simulink model "QPSK_TX_Final"  (R2017b)
settings: Solver=FixedStepDiscrete  StartTime=0.0  StopTime=1  RelTol=1e-3
PreLoadFcn:
  | qpsktxhdl=QPSK_final_init;
libraries: hdlsllib x3, dspmlti4 x2, commdigbbndpm3 x1
settings Model: DataTypeOverride=Off  Creator=The MathWorks, Inc.  LastModifiedBy=ppradhan
settings DataIOCC: LimitDataPoints=on  SaveFormat=Array  SaveOutput=off  SaveTime=off
settings OptimizationCC: BlockReduction=off  ConditionallyExecuteInputs=off  DefaultParameterBehavior=Inlined  LifeSpan=inf
settings DebuggingCC: AlgebraicLoopMsg=error  UnderspecifiedInitializationDetection=Classic  MergeDetectMultiDrivingBlocksExec=none  SolverPrmCheckMsg=warning  MultiTaskDSMMsg=warning  MultiTaskCondExecSysMsg=none  SingleTaskRateTransMsg=error  IntegerOverflowMsg=none  ParameterPrecisionLossMsg=none  AllowSymbolicDim=off  StateNameClashWarn=warning  SFUnexpectedBacktrackingDiag=warning  SFNoUnconditionalDefaultTransitionDiag=warning  SFExecutionAtInitializationDiag=none  IntegerSaturationMsg=none
settings HardwareCC: ProdBitPerPointer=32  ProdBitPerSizeT=32  ProdBitPerPtrDiffT=32  ProdLargestAtomicFloat=None  ProdIntDivRoundTo=Undefined  ProdEndianess=Unspecified  ProdWordSize=32  ProdHWDeviceType=ASIC/FPGA->ASIC/FPGA  ProdEqTarget=off
settings ModelReferenceCC: PropagateSignalLabelsOutOfModel=off
settings CodeAppCC: StateflowObjectComments=on
settings GRTTargetCC: TargetLangStandard=C89/C90 (ANSI)  GeneratePreprocessorConditionals=Disable all
settings ConfigComp: CovMetricSettings=dw  CovHtmlReporting=on  CovSaveCumulativeToWorkspaceVar=on  CovSaveSingleToWorkspaceVar=on  CovExternalEMLEnable=off  CovSFcnEnable=off

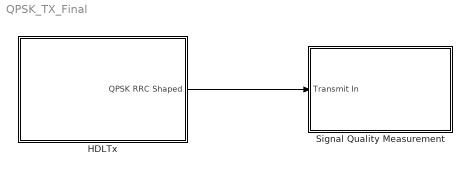
== system QPSK_TX_Final ==
  HDLTx : Subsystem
  Signal Quality Measurement : Subsystem
  wires:
  HDLTx/1(QPSK RRC Shaped) -> Signal Quality Measurement/1(Transmit In)

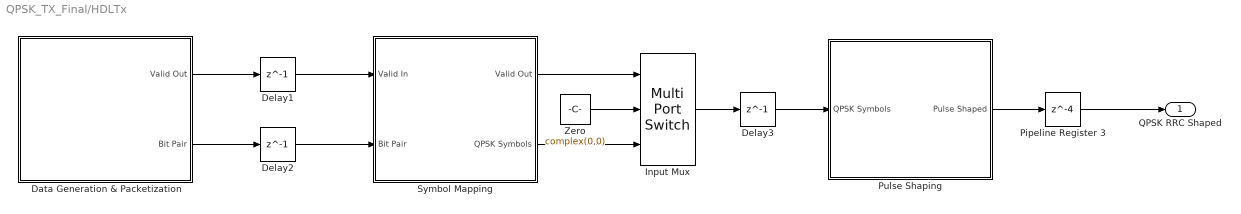
== system QPSK_TX_Final/HDLTx ==
  " Zero" : Constant  Value=complex(0,0)  OutDataTypeStr=fixdt(1,16,15)  SampleTime=(qpsktxhdl.Ts)*4
  Data Generation & Packetization : Subsystem
  Delay1 : Delay  DelayLength=1  InitialCondition=0
  Delay2 : Delay  DelayLength=1  InitialCondition=0
  Delay3 : Delay  DelayLength=1  InitialCondition=0
  Input Mux : MultiPortSwitch  DataPortOrder=Zero-based contiguous  Inputs=2
  Pipeline Register 3 : Delay  DelayLength=4  InitialCondition=0
  Pulse Shaping : Subsystem
  Symbol Mapping : Subsystem
  QPSK RRC Shaped : Outport
  wires:
  " Zero"/1 -> Input Mux/2
  Symbol Mapping/2(QPSK Symbols) -> Input Mux/3
  Symbol Mapping/1(Valid Out) -> Input Mux/1
  Delay3/1 -> Pulse Shaping/1(QPSK Symbols)
  Input Mux/1 -> Delay3/1
  Delay1/1 -> Symbol Mapping/1(Valid In)
  Pulse Shaping/1(Pulse Shaped) -> Pipeline Register 3/1
  Data Generation & Packetization/1(Valid Out) -> Delay1/1
  Pipeline Register 3/1 -> QPSK RRC Shaped/1
  Data Generation & Packetization/2(Bit Pair) -> Delay2/1
  Delay2/1 -> Symbol Mapping/2(Bit Pair)

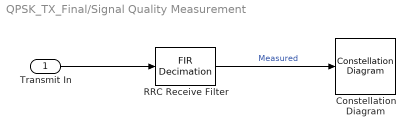
== system QPSK_TX_Final/Signal Quality Measurement ==
  Transmit In : Inport
  Constellation Diagram : ConstellationDiagram
  RRC Receive Filter : dspmlti4/FIR Decimation  FilterSource=Dialog parameters  h=qpsktxhdl.rcRxFilt  D=qpsktxhdl.Upsampling  filtStruct=Direct form  FilterObject=Hm_firdecim  framing=Allow multirate processing  inputOffset=0  outputBufInitCond=0  roundingMode=Floor  overflowMode=off  firstCoeffMode=Binary point scaling  firstCoeffWordLength=16  firstCoeffFracLength=15  firstCoeffDataTypeStr=fixdt(1,16,15)  firstCoeffMin=[]  firstCoeffMax=[]  firstCoeffLastDataTypeStr=fixdt(1,16,15)  prodOutputMode=Binary point scaling  prodOutputWordLength=32  prodOutputFracLength=30  prodOutputDataTypeStr=fixdt(1,32,30)  prodOutputLastDataTypeStr=fixdt(1,32,30)  accumMode=Binary point scaling  accumWordLength=33  accumFracLength=30  accumDataTypeStr=fixdt(1,33,30)  accumLastDataTypeStr=fixdt(1,33,30)  outputMode=Binary point scaling  outputWordLength=33  outputFracLength=30  outputDataTypeStr=fixdt(1,33,30)  outputMin=[]  outputMax=[]  outputLastDataTypeStr=fixdt(1,33,30)
  wires:
  Transmit In/1 -> RRC Receive Filter/1
  RRC Receive Filter/1 -> Constellation Diagram/1  "Measured"

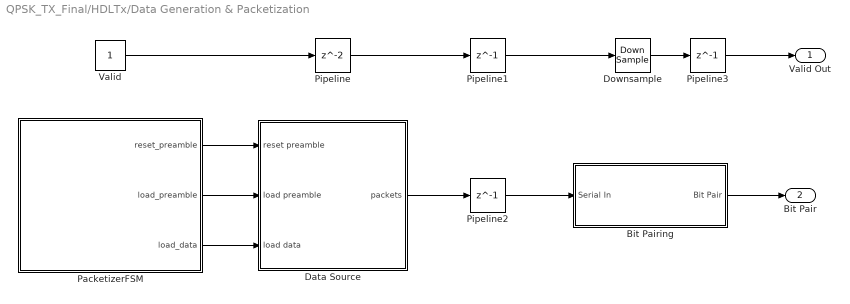
== system QPSK_TX_Final/HDLTx/Data Generation & Packetization ==
  Bit Pairing : Subsystem
  Data Source : Subsystem
  Downsample : DownSample  RateOptions=Allow multirate processing
  PacketizerFSM : MATLAB Function  TreatAsAtomicUnit=on  SystemSampleTime=(qpsktxhdl.Ts)*2
  Pipeline : Delay  InitialCondition=0
  Pipeline1 : Delay  DelayLength=1  InitialCondition=0
  Pipeline2 : Delay  DelayLength=1  InitialCondition=0
  Pipeline3 : Delay  DelayLength=1  InitialCondition=0
  Valid : Constant  OutDataTypeStr=boolean  SampleTime=(qpsktxhdl.Ts)*2
  Valid Out : Outport
  Bit Pair : Outport  Port=2
  wires:
  Bit Pairing/1(Bit Pair) -> Bit Pair/1
  Pipeline2/1 -> Bit Pairing/1(Serial In)
  Data Source/1(packets) -> Pipeline2/1
  Valid/1 -> Pipeline/1
  Pipeline1/1 -> Downsample/1
  Pipeline/1 -> Pipeline1/1
  Downsample/1 -> Pipeline3/1
  Pipeline3/1 -> Valid Out/1
  PacketizerFSM/1(reset_preamble) -> Data Source/1(reset preamble)
  PacketizerFSM/2(load_preamble) -> Data Source/2(load preamble)
  PacketizerFSM/3(load_data) -> Data Source/3(load data)

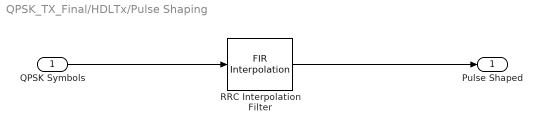
== system QPSK_TX_Final/HDLTx/Pulse Shaping ==
  QPSK Symbols : Inport
  RRC Interpolation Filter : dspmlti4/FIR Interpolation  FilterSource=Dialog parameters  h=qpsktxhdl.rcTxFilt  L=qpsktxhdl.Upsampling  FilterObject=Htxrc  framing=Allow multirate processing  outputBufInitCond=0  roundingMode=Floor  overflowMode=off  firstCoeffMode=Binary point scaling  firstCoeffWordLength=16  firstCoeffFracLength=15  firstCoeffDataTypeStr=fixdt(1,16,15)  firstCoeffMin=[]  firstCoeffMax=[]  firstCoeffLastDataTypeStr=fixdt(1,16,15)  prodOutputMode=Binary point scaling  prodOutputWordLength=16  prodOutputFracLength=15  prodOutputDataTypeStr=fixdt(1,16,15)  prodOutputLastDataTypeStr=fixdt(1,16,15)  accumMode=Binary point scaling  accumWordLength=16  accumFracLength=15  accumDataTypeStr=fixdt(1,16,15)  accumLastDataTypeStr=fixdt(1,16,15)  outputMode=Binary point scaling  outputWordLength=16  outputFracLength=15  outputDataTypeStr=fixdt(1,16,15)  outputMin=[]  outputMax=[]  outputLastDataTypeStr=fixdt(1,16,15)
      settings: SourceProductName=DSP System Toolbox
  Pulse Shaped : Outport
  wires:
  RRC Interpolation Filter/1 -> Pulse Shaped/1
  QPSK Symbols/1 -> RRC Interpolation Filter/1

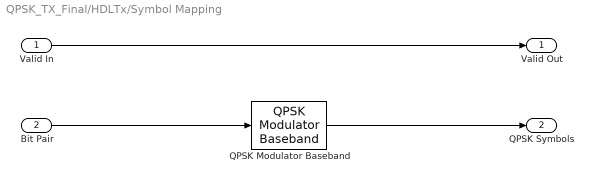
== system QPSK_TX_Final/HDLTx/Symbol Mapping ==
  Valid In : Inport
  Bit Pair : Inport  Port=2
  QPSK Modulator Baseband : commdigbbndpm3/QPSK Modulator Baseband  InType=Integer  Enc=Gray  Ph=pi/4  outDtype=Fixed-point  outWordLen=2  outUDDataType=sfix(16)  outFracLenMode=User-defined  outFracLen=0  outDataTypeStr=fixdt(1,2,0)  outLastDataTypeStr=fixdt(1,2,0)
  Valid Out : Outport
  QPSK Symbols : Outport  Port=2
  wires:
  Valid In/1 -> Valid Out/1
  Bit Pair/1 -> QPSK Modulator Baseband/1
  QPSK Modulator Baseband/1 -> QPSK Symbols/1

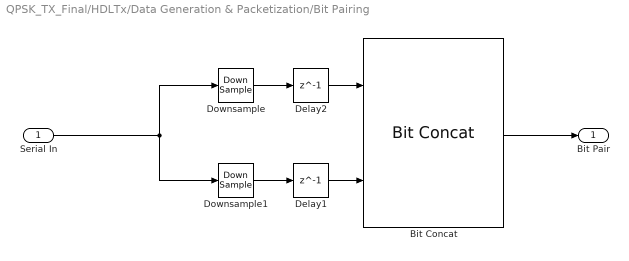
== system QPSK_TX_Final/HDLTx/Data Generation & Packetization/Bit Pairing ==
  Serial In : Inport
  Bit Concat : hdlsllib/HDL Operations/Bit Concat  numInputs=2
      settings: SourceProductName=HDL Coder  SourceProductBaseCode=HD
  Delay1 : Delay  DelayLength=1
  Delay2 : Delay  DelayLength=1
  Downsample : DownSample  phase=1  RateOptions=Allow multirate processing
  Downsample1 : DownSample  RateOptions=Allow multirate processing
  Bit Pair : Outport
  wires:
  Downsample1/1 -> Delay1/1
  Serial In/1 -> Downsample1/1, Downsample/1
  Bit Concat/1 -> Bit Pair/1
  Downsample/1 -> Delay2/1
  Delay1/1 -> Bit Concat/2
  Delay2/1 -> Bit Concat/1

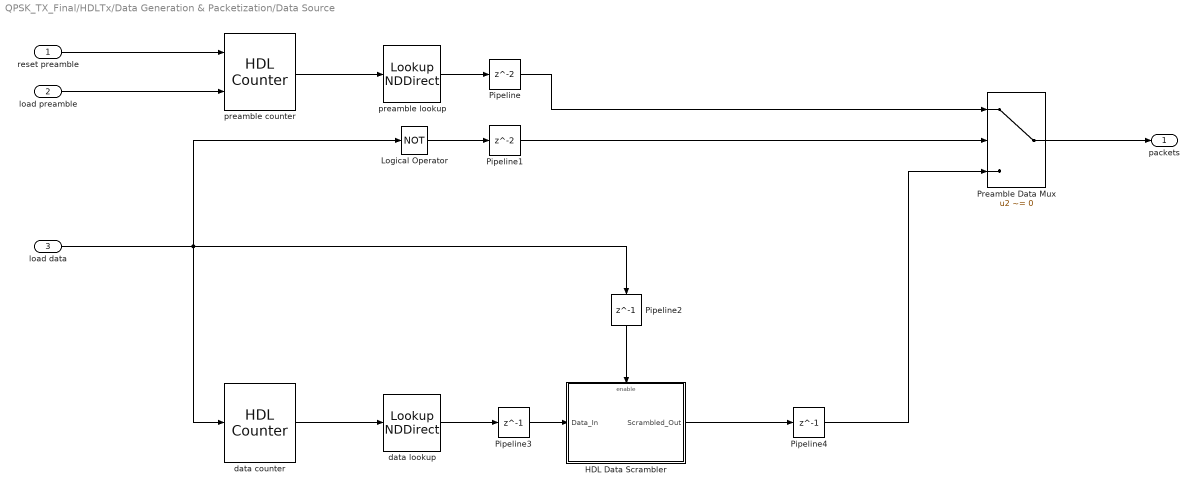
== system QPSK_TX_Final/HDLTx/Data Generation & Packetization/Data Source ==
  reset preamble : Inport
  load preamble : Inport  Port=2
  load data : Inport  Port=3
  HDL Data Scrambler : Subsystem  TreatAsAtomicUnit=on
  Logical Operator : Logic  Operator=NOT  AllPortsSameDT=off  OutDataTypeStr=boolean
  Pipeline : Delay  InitialCondition=0
  Pipeline1 : Delay  InitialCondition=0
  Pipeline2 : Delay  DelayLength=1  InitialCondition=0
  Pipeline3 : Delay  DelayLength=1  InitialCondition=0
  Pipeline4 : Delay  DelayLength=1  InitialCondition=0
  Preamble Data Mux : Switch  Criteria=u2 ~= 0
  data counter : hdlsllib/HDL Operations/HDL Counter  CountType=Count limited  CountInit=0  CountStep=1  CountMax=17399  CountFromType=Initial value  CountFrom=0  CountResetPort=off  CountLoadPort=off  CountEnbPort=on  CountDirPort=off  CountDataType=Unsigned  CountWordLen=16  CountFracLen=0  CountSampTime=1
      settings: SourceProductName=HDL Coder  SourceProductBaseCode=HD
  data lookup : LookupNDDirect  NumberOfTableDimensions=1  Table=[qpsktxhdl.data]  DiagnosticForOutOfRangeInput=Error  TableDataTypeStr=boolean
  preamble counter : hdlsllib/HDL Operations/HDL Counter  CountType=Free running  CountInit=0  CountStep=1  CountMax=256  CountFromType=Initial value  CountFrom=0  CountResetPort=on  CountLoadPort=off  CountEnbPort=on  CountDirPort=off  CountDataType=Unsigned  CountWordLen=8  CountFracLen=0  CountSampTime=1
      settings: SourceProductName=HDL Coder  SourceProductBaseCode=HD
  preamble lookup : LookupNDDirect  NumberOfTableDimensions=1  Table=[qpsktxhdl.preamble]  DiagnosticForOutOfRangeInput=Error  TableDataTypeStr=boolean
  packets : Outport
  wires:
  load data/1 -> Pipeline2/1, Logical Operator/1, data counter/1
  Logical Operator/1 -> Pipeline1/1
  Pipeline2/1 -> HDL Data Scrambler/Enable
  Preamble Data Mux/1 -> packets/1
  Pipeline1/1 -> Preamble Data Mux/2
  Pipeline/1 -> Preamble Data Mux/1
  Pipeline4/1 -> Preamble Data Mux/3
  Pipeline3/1 -> HDL Data Scrambler/1(Data_In)
  preamble lookup/1 -> Pipeline/1
  HDL Data Scrambler/1(Scrambled_Out) -> Pipeline4/1
  data lookup/1 -> Pipeline3/1
  data counter/1 -> data lookup/1
  reset preamble/1 -> preamble counter/1
  load preamble/1 -> preamble counter/2
  preamble counter/1 -> preamble lookup/1

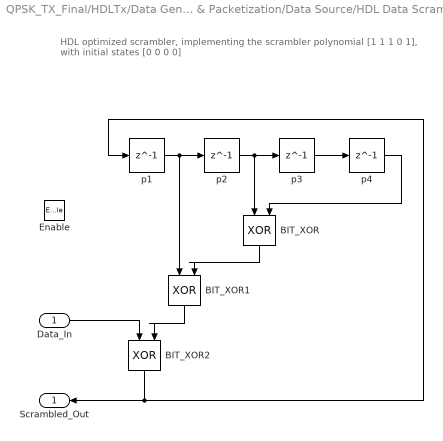
== system QPSK_TX_Final/HDLTx/Data Generation & Packetization/Data Source/HDL Data Scrambler ==
  note: HDL optimized scrambler, implementing the scrambler
      | polynomial [1 1 1 0 1], with initial states [0 0 0 0]
  Data_In : Inport
  Enable : EnablePort
  BIT_XOR : Logic  Operator=XOR  IconShape=distinctive  AllPortsSameDT=off  OutDataTypeStr=boolean
  BIT_XOR1 : Logic  Operator=XOR  IconShape=distinctive  AllPortsSameDT=off  OutDataTypeStr=boolean
  BIT_XOR2 : Logic  Operator=XOR  IconShape=distinctive  AllPortsSameDT=off  OutDataTypeStr=boolean
  p{1..4} (4 alike) : Delay  DelayLength=1
  Scrambled_Out : Outport  InitialOutput=0
  wires:
  BIT_XOR2/1 -> p1/1, Scrambled_Out/1
  p4/1 -> BIT_XOR/2
  p1/1 -> p2/1, BIT_XOR1/1
  BIT_XOR/1 -> BIT_XOR1/2
  p3/1 -> p4/1
  p2/1 -> p3/1, BIT_XOR/1
  BIT_XOR1/1 -> BIT_XOR2/2
  Data_In/1 -> BIT_XOR2/1

== matlab function QPSK_TX_Final/HDLTx/Data Generation & Packetization/PacketizerFSM ==
  data: reset_preamble output; load_preamble output; load_data output
function [reset_preamble,load_preamble, load_data] = PacketizerFSM()
%#codegen

persistent packState;
persistent stateCounter;

sType = numerictype(0,1,0);
cType = numerictype(0,8,0);

if isempty(packState)
    packState = fi(0,'numerictype',sType);
    stateCounter  = fi(0,'numerictype',cType);
end

Pack_Preamble = fi(0,'numerictype',sType);
Append_Data   = fi(1,'numerictype',sType);

switch(packState)
    case Pack_Preamble %% Pack_Preamble
        load_preamble  = true;
        reset_preamble = false;
        load_data     = false;
        
        if stateCounter == 25; %% preamble loaded
            packState(:) = 1;      %% move to data packing
            stateCounter(:) = 0;   %% reset counter
        else
            packState(:) = 0;      %% remain in preamble packing
            stateCounter(:) = stateCounter +1; %% increment preamble count
        end
        
    case Append_Data %% Append_Data
        load_preamble  = false;
        reset_preamble = true;
        load_data     = true;
        
        if stateCounter == 173 %% data loaded
            packState(:) = 0;      %% move to preamble packing
            stateCounter(:) = 0;   %% reset counter
        else
            packState(:) = 1;      %% remain in data loading
            stateCounter(:) = stateCounter +1; %% increment data count
        end
        
    otherwise
        load_preamble  = false;
        reset_preamble = false;
        load_data     = false;
        stateCounter(:) = 0;
end
